simulink model "rThrottle"  (R2024b)
settings: Solver=FixedStepDiscrete  StartTime=0.0  StopTime=1  FixedStep=0.001  RelTol=1e-3  EnableMultiTasking=on
undefined symbols (not defined in the file): rThrottlePedal1Gain, rThrottlePedal2Gain
settings Model: DataDictionary=Master_Dictionary.sldd  EnableAccessToBaseWorkspace=off  Creator=torni  LastModifiedBy=oxbro
settings SolverCC: AlgebraicLoopSolver=TrustRegion
settings DataIOCC: ReturnWorkspaceOutputs=off
settings OptimizationCC: DefaultParameterBehavior=Inlined  EnhancedBackFolding=on  PassReuseOutputArgsAs=Individual arguments  ZeroExternalMemoryAtStartup=off  ZeroInternalMemoryAtStartup=off  MaxStackSize=512  OptimizeBlockOrder=speed  DifferentSizesBufferReuse=on  OptimizationCustomize=off  EfficientTunableParamExpr=on
settings DebuggingCC: ParameterTunabilityLossMsg=error  UnconnectedInputMsg=warning  UnconnectedOutputMsg=warning  UnconnectedLineMsg=warning  ArithmeticOperatorsInVariantConditions=warning
settings HardwareCC: ProdBitPerPointer=32  ProdBitPerSizeT=32  ProdBitPerPtrDiffT=32  ProdLargestAtomicInteger=Long  ProdLargestAtomicFloat=Double  ProdWordSize=32  ProdLongLongMode=on  ProdHWDeviceType=ARM Compatible->ARM Cortex-M
settings ModelReferenceCC: EnableRefExpFcnMdlSchedulingChecks=on
settings SFSimCC: MATLABDynamicMemAlloc=off  CustomCodeUndefinedFunction=UseInterfaceOnly
settings RTWCC: Description=Embedded Coder  SystemTargetFile=ert.tlc  HardwareBoard=STM32H7xx Based (Single-core)  TemplateMakefile=ert_default_tmf  CustomHeaderCode="#include \"stm32h7xx_ll_tim.h\""  CustomInitializer=LL_TIM_EnableCounter(TIM2);  Toolchain=GNU Tools for ARM Embedded Processors  GPUComputeCapability=3.5
settings CodeAppCC: ForceParamTrailComments=on  IgnoreCustomStorageClasses=off  OperatorAnnotations=on  SimulinkDataObjDesc=on  SFDataObjDesc=on  InsertBlockDesc=on
settings ERTTargetCC: TargetLangStandard=C99 (ISO)  CodeReplacementLibrary=ARM Cortex-M  ExtModeTransport=3  ExtModeStaticAlloc=on  ExtModeStaticAllocSize=2048  ExtModeMexFile=ext_xcp  ExtModeIntrfLevel=Level2 - Open

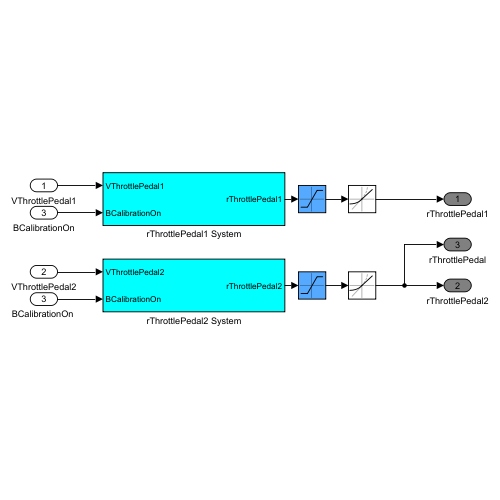
[thumbnail: Simulink's stored preview of the top-level diagram]
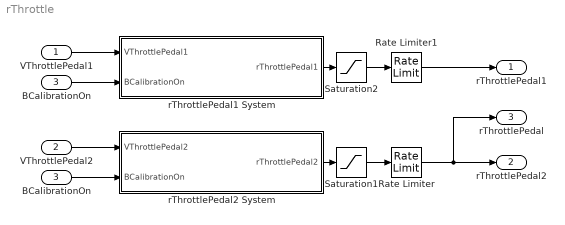
== system rThrottle ==
  VThrottlePedal1 : Inport  OutDataTypeStr=double
  VThrottlePedal2 : Inport  Port=2  OutDataTypeStr=double
  BCalibrationOn : Inport  Port=3  OutDataTypeStr=boolean
  "BCalibrationOn " : InportShadow  Port=3  OutDataTypeStr=boolean
  Rate Limiter : RateLimiter  RisingSlewLimit=375  FallingSlewLimit=-1000  SampleTimeMode=inherited
  Rate Limiter1 : RateLimiter  RisingSlewLimit=375  FallingSlewLimit=-1000  SampleTimeMode=inherited
  Saturation1 : Saturate  UpperLimit=100  LowerLimit=0
  Saturation2 : Saturate  UpperLimit=100  LowerLimit=0
  rThrottlePedal1 System : Subsystem
  rThrottlePedal2 System : Subsystem
  rThrottlePedal1 : Outport  OutDataTypeStr=double  VectorParamsAs1DForOutWhenUnconnected=off
  rThrottlePedal2 : Outport  Port=2  OutDataTypeStr=double  VectorParamsAs1DForOutWhenUnconnected=off
  rThrottlePedal : Outport  Port=3  OutDataTypeStr=double  VectorParamsAs1DForOutWhenUnconnected=off
  wires:
  rThrottlePedal1 System/1(rThrottlePedal1) -> Saturation2/1
  VThrottlePedal1/1 -> rThrottlePedal1 System/1(VThrottlePedal1)
  VThrottlePedal2/1 -> rThrottlePedal2 System/1(VThrottlePedal2)
  rThrottlePedal2 System/1(rThrottlePedal2) -> Saturation1/1
  Saturation2/1 -> Rate Limiter1/1
  Saturation1/1 -> Rate Limiter/1
  "BCalibrationOn "/1 -> rThrottlePedal2 System/2(BCalibrationOn)
  BCalibrationOn/1 -> rThrottlePedal1 System/2(BCalibrationOn)
  Rate Limiter/1 -> rThrottlePedal2/1, rThrottlePedal/1
  Rate Limiter1/1 -> rThrottlePedal1/1

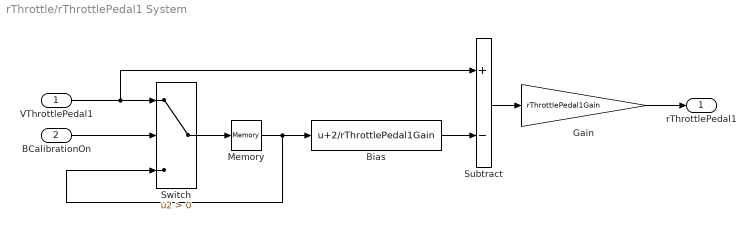
== system rThrottle/rThrottlePedal1 System ==
  VThrottlePedal1 : Inport  OutDataTypeStr=double
  BCalibrationOn : Inport  Port=2  OutDataTypeStr=boolean
  Bias : Bias  Bias=2/rThrottlePedal1Gain  SaturateOnIntegerOverflow=off
  Gain : Gain  Gain=rThrottlePedal1Gain  OutDataTypeStr=double
  Memory : Memory  InheritSampleTime=on
  Subtract : Sum  Inputs=+-
  Switch : Switch  Criteria=u2 > Threshold  SaturateOnIntegerOverflow=off  InputSameDT=off
  rThrottlePedal1 : Outport  OutDataTypeStr=double  VectorParamsAs1DForOutWhenUnconnected=off
  wires:
  VThrottlePedal1/1 -> Subtract/1, Switch/1
  BCalibrationOn/1 -> Switch/2
  Switch/1 -> Memory/1
  Memory/1 -> Switch/3, Bias/1
  Subtract/1 -> Gain/1
  Bias/1 -> Subtract/2
  Gain/1 -> rThrottlePedal1/1

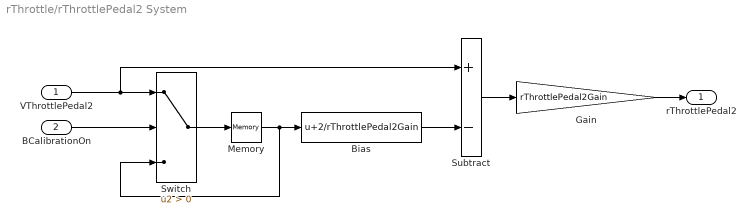
== system rThrottle/rThrottlePedal2 System ==
  VThrottlePedal2 : Inport  OutDataTypeStr=double
  BCalibrationOn : Inport  Port=2  OutDataTypeStr=boolean
  Bias : Bias  Bias=2/rThrottlePedal2Gain  SaturateOnIntegerOverflow=off
  Gain : Gain  Gain=rThrottlePedal2Gain  OutDataTypeStr=double
  Memory : Memory  InheritSampleTime=on
  Subtract : Sum  Inputs=+-
  Switch : Switch  Criteria=u2 > Threshold  SaturateOnIntegerOverflow=off  InputSameDT=off
  rThrottlePedal2 : Outport  OutDataTypeStr=double  VectorParamsAs1DForOutWhenUnconnected=off
  wires:
  VThrottlePedal2/1 -> Subtract/1, Switch/1
  BCalibrationOn/1 -> Switch/2
  Switch/1 -> Memory/1
  Memory/1 -> Switch/3, Bias/1
  Bias/1 -> Subtract/2
  Subtract/1 -> Gain/1
  Gain/1 -> rThrottlePedal2/1
